simulink model "MCity_cs"  (Simulink 8.9)
settings: Solver=ode5  StartTime=0.0  StopTime=2.95  FixedStep=1/200  RelTol=1e-3
PreLoadFcn:
  | check_NUTS_defined;
  | 
  | assignin('base',['model_closed_' bdroot],false);
InitFcn:
  | PreScanExperimentInitFcn(bdroot)
StopFcn:
  | PreScanExperimentStopFcn(bdroot)
values from neighbouring files (symbols this model uses):
  d_offset = -18.15    [monocityTestLeftTurn.mat]    (also in simulation_leftTurn_PreScan.m = dl/vl*vh - 43 + R)
undefined symbols (not defined in the file or in its folder): DiscIntNeverNeededParam, warningInitialVelocity, x0
libraries: simulink x73, PreScanSimulinkLibrary x14, simulink_extras x10, PreScanUsefulBlocks x4
(part 9 of 11)

== system MCity_cs/BMW_Z3_1/Dynamics_Simple/Chassis/Bicycle_model_[XYZ]/Y & Yaw_Motion ==
  |vx|_[ms-1] : Inport
  Fy_[N] : Inport  Port=2
  Mz_[Nm] : Inport  Port=3
  Compare To Zero : simulink/Logic and Bit Operations/Compare To Zero  relop===  OutDataTypeStr=boolean  ZeroCross=off
  Configurable Subsystem : Subsystem  BlockChoice=Integrator  mask{ComputationMode=ComputationMode}
      mask prompts: ComputationMode "Computation mode:"
      mask init:
      | SetComputationMode(gcb,ComputationMode);
      settings: AttributesFormatString=%<BlockChoice>  OpenFcn=BringToFront(gcb);  MemberBlocks=Discrete-Time Integrator,Integrator
      settings: TemplateBlock=|
      | PreScanSimulinkLibrary/Configurable Subsystems/integral with reset/Configurable
      | Subsystem
  Configurable Subsystem1 : Subsystem  BlockChoice=Integrator  mask{ComputationMode=ComputationMode}
      link override Discrete-Time Integrator: IntegratorMethod=Integration: Backward Euler
      mask prompts: ComputationMode "Computation mode:"
      mask init:
      | SetComputationMode(gcb,ComputationMode);
      settings: AttributesFormatString=%<BlockChoice>  OpenFcn=BringToFront(gcb);  MemberBlocks=Discrete-Time Integrator,Integrator
      settings: TemplateBlock=|
      | PreScanSimulinkLibrary/Configurable Subsystems/integral/Configurable
      | Subsystem1
  Configurable Subsystem2 : Subsystem  BlockChoice=Integrator  mask{ComputationMode=ComputationMode}
      mask prompts: ComputationMode "Computation mode:"
      mask init:
      | SetComputationMode(gcb,ComputationMode);
      settings: AttributesFormatString=%<BlockChoice>  OpenFcn=BringToFront(gcb);  MemberBlocks=Discrete-Time Integrator,Integrator
      settings: TemplateBlock=|
      | PreScanSimulinkLibrary/Configurable Subsystems/integral with reset/Configurable
      | Subsystem
  Fcn1 : Fcn  Expr=u(1)*u(3)
  Gain : Gain  Gain=1/p.m  SaturateOnIntegerOverflow=on  OutDataTypeStr=Inherit: Same as input  ParamDataTypeStr=Inherit: Same as input
  Gain1 : Gain  Gain=1/p.J_zz  SaturateOnIntegerOverflow=on  OutDataTypeStr=Inherit: Same as input  ParamDataTypeStr=Inherit: Same as input
  Sum1 : Sum  Inputs=-+  SaturateOnIntegerOverflow=on  InputSameDT=on  OutDataTypeStr=Inherit: Same as first input
  mux : Mux  Inputs=3
  |vx|_[ms-1]1 : Outport  InitialOutput=0
  vy_[ms-1] : Outport  Port=2  InitialOutput=0
  ay_[ms-2] : Outport  Port=3  InitialOutput=0
  dYawAngle_[rads-1] : Outport  Port=4  InitialOutput=0
  YawAngle_[rad] : Outport  Port=5  InitialOutput=0
  wires:
  Configurable Subsystem2/1(Out1) -> Configurable Subsystem1/1(In1), mux/3, dYawAngle_[rads-1]/1  "dYawAngle_[rads-1]"
  Configurable Subsystem/1(Out1) -> mux/2, vy_[ms-1]/1  "vy_[ms-1]"
  |vx|_[ms-1]/1 -> mux/1, |vx|_[ms-1]1/1, Compare To Zero/1  "|vx|_[ms-1]"
  mux/1 -> Fcn1/1  "|vx|_[ms-1]_vy_[ms-1]_dYawAngle_[rads-1]"
  Fcn1/1 -> Sum1/1  "|vx|*dYawAngle_[ms-2]"
  Sum1/1 -> Configurable Subsystem/1(In1)  "dvy_[ms-2]"
  Fy_[N]/1 -> Gain/1  "Fy_[N]"
  Mz_[Nm]/1 -> Gain1/1  "Mz_[Nm]"
  Configurable Subsystem1/1(Out1) -> YawAngle_[rad]/1
  Compare To Zero/1 -> [reset]
  [reset] -> Configurable Subsystem2/2(In2)
  [reset] -> Configurable Subsystem/2(In2)
  Gain/1 -> ay_[ms-2]/1, Sum1/2  "ddy_[ms-2]"
  Gain1/1 -> Configurable Subsystem2/1(In1)  "ddYawAngle_[rads-2]"

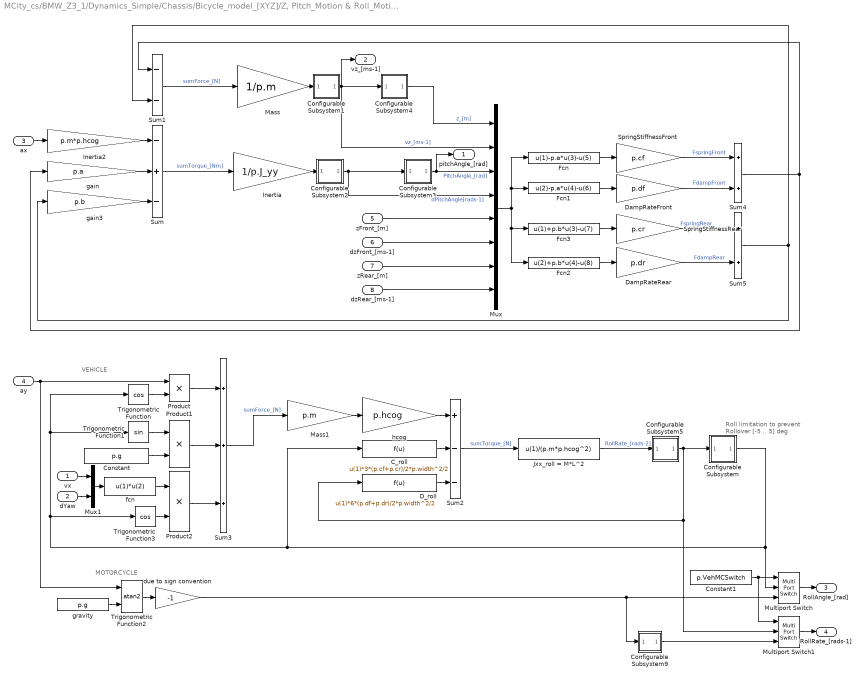
== system MCity_cs/BMW_Z3_1/Dynamics_Simple/Chassis/Bicycle_model_[XYZ]/Z, Pitch_Motion & Roll_Motion ==
  note: MOTORCYCLE
  note: VEHICLE
  note: Roll limitation
      | to prevent
      | Rollover
      | [-5 .. 5] deg
  vx : Inport
  dYaw : Inport  Port=2
  ax : Inport  Port=3
  ay : Inport  Port=4
  zFront_[m] : Inport  Port=5
  dzFront_[ms-1] : Inport  Port=6
  zRear_[m] : Inport  Port=7
  dzRear_[ms-1] : Inport  Port=8
  C_roll : Fcn  Expr=u(1)*3*(p.cf+p.cr)/2*p.width^2/2
  Configurable Subsystem : Subsystem  BlockChoice=Integrator  mask{ComputationMode=ComputationMode}
      link override Discrete-Time Integrator: UpperSaturationLimit=5*pi/180  LowerSaturationLimit=-5*pi/180
      link override Integrator: UpperSaturationLimit=5*pi/180  LowerSaturationLimit=-5*pi/180
      mask prompts: ComputationMode "Computation mode:"
      mask init:
      | SetComputationMode(gcb,ComputationMode);
      settings: AttributesFormatString=%<BlockChoice>  OpenFcn=BringToFront(gcb);  MemberBlocks=Discrete-Time Integrator,Integrator
      settings: TemplateBlock=|
      | PreScanSimulinkLibrary/Configurable Subsystems/integral with limits
      | for roll motion/Configurable
      | Subsystem
  Configurable Subsystem1 : Subsystem  BlockChoice=Integrator  mask{ComputationMode=ComputationMode}
      mask prompts: ComputationMode "Computation mode:"
      mask init:
      | SetComputationMode(gcb,ComputationMode);
      settings: AttributesFormatString=%<BlockChoice>  OpenFcn=BringToFront(gcb);  MemberBlocks=Discrete-Time Integrator,Integrator
      settings: TemplateBlock=|
      | PreScanSimulinkLibrary/Configurable Subsystems/integral/Configurable
      | Subsystem1
  Configurable Subsystem2 : Subsystem  BlockChoice=Integrator  mask{ComputationMode=ComputationMode}
      mask prompts: ComputationMode "Computation mode:"
      mask init:
      | SetComputationMode(gcb,ComputationMode);
      settings: AttributesFormatString=%<BlockChoice>  OpenFcn=BringToFront(gcb);  MemberBlocks=Discrete-Time Integrator,Integrator
      settings: TemplateBlock=|
      | PreScanSimulinkLibrary/Configurable Subsystems/integral/Configurable
      | Subsystem1
  Configurable Subsystem3 : Subsystem  BlockChoice=Integrator  mask{ComputationMode=ComputationMode}
      mask prompts: ComputationMode "Computation mode:"
      mask init:
      | SetComputationMode(gcb,ComputationMode);
      settings: AttributesFormatString=%<BlockChoice>  OpenFcn=BringToFront(gcb);  MemberBlocks=Discrete-Time Integrator,Integrator
      settings: TemplateBlock=|
      | PreScanSimulinkLibrary/Configurable Subsystems/integral/Configurable
      | Subsystem1
  Configurable Subsystem4 : Subsystem  BlockChoice=Integrator  mask{ComputationMode=ComputationMode}
      mask prompts: ComputationMode "Computation mode:"
      mask init:
      | SetComputationMode(gcb,ComputationMode);
      settings: AttributesFormatString=%<BlockChoice>  OpenFcn=BringToFront(gcb);  MemberBlocks=Discrete-Time Integrator,Integrator
      settings: TemplateBlock=|
      | PreScanSimulinkLibrary/Configurable Subsystems/integral/Configurable
      | Subsystem1
  Configurable Subsystem5 : Subsystem  BlockChoice=Integrator  mask{ComputationMode=ComputationMode}
      mask prompts: ComputationMode "Computation mode:"
      mask init:
      | SetComputationMode(gcb,ComputationMode);
      settings: AttributesFormatString=%<BlockChoice>  OpenFcn=BringToFront(gcb);  MemberBlocks=Discrete-Time Integrator,Integrator
      settings: TemplateBlock=|
      | PreScanSimulinkLibrary/Configurable Subsystems/integral/Configurable
      | Subsystem1
  Configurable Subsystem9 : Subsystem  BlockChoice=Derivative  mask{ComputationMode=ComputationMode}
      mask prompts: ComputationMode "Computation mode:"
      mask init:
      | SetComputationMode(gcb,ComputationMode);
      settings: AttributesFormatString=%<BlockChoice>  OpenFcn=BringToFront(gcb);  MemberBlocks=Derivative,Discrete Derivative
      settings: TemplateBlock=|
      | PreScanSimulinkLibrary/Configurable Subsystems/Derivative/Configurable
      | Subsystem
  Constant : Constant  Value=p.g
  Constant1 : Constant  Value=p.VehMCSwitch
  D_roll : Fcn  Expr=u(1)*6*(p.df+p.dr)/2*p.width^2/2
  DampRateFront : Gain  Gain=p.df  SaturateOnIntegerOverflow=on  OutDataTypeStr=Inherit: Same as input  ParamDataTypeStr=Inherit: Same as input
  DampRateRear : Gain  Gain=p.dr  SaturateOnIntegerOverflow=on  OutDataTypeStr=Inherit: Same as input  ParamDataTypeStr=Inherit: Same as input
  Fcn : Fcn  Expr=u(1)-p.a*u(3)-u(5)
  Fcn1 : Fcn  Expr=u(2)-p.a*u(4)-u(6)
  Fcn2 : Fcn  Expr=u(2)+p.b*u(4)-u(8)
  Fcn3 : Fcn  Expr=u(1)+p.b*u(3)-u(7)
  Inertia : Gain  Gain=1/p.J_yy  SaturateOnIntegerOverflow=on  OutDataTypeStr=Inherit: Same as input  ParamDataTypeStr=Inherit: Same as input
  Inertia2 : Gain  Gain=p.m*p.hcog  SaturateOnIntegerOverflow=on  OutDataTypeStr=Inherit: Same as input  ParamDataTypeStr=Inherit: Same as input
  Jxx_roll = M*L^2 : Fcn  Expr=u(1)/(p.m*p.hcog^2)
  Mass : Gain  Gain=1/p.m  SaturateOnIntegerOverflow=on  OutDataTypeStr=Inherit: Same as input  ParamDataTypeStr=Inherit: Same as input
  Mass1 : Gain  Gain=p.m  SaturateOnIntegerOverflow=on  OutDataTypeStr=Inherit: Same as input  ParamDataTypeStr=Inherit: Same as input
  Multiport Switch : MultiPortSwitch  Inputs=2
  Multiport Switch1 : MultiPortSwitch  Inputs=2
  Mux : Mux  Inputs=8
  Mux1 : Mux  Inputs=2
  Product : Product  RndMeth=Zero
  Product1 : Product  RndMeth=Zero
  Product2 : Product  RndMeth=Zero
  SpringStiffnessFront : Gain  Gain=p.cf  SaturateOnIntegerOverflow=on  OutDataTypeStr=Inherit: Same as input  ParamDataTypeStr=Inherit: Same as input
  SpringStiffnessRear : Gain  Gain=p.cr  SaturateOnIntegerOverflow=on  OutDataTypeStr=Inherit: Same as input  ParamDataTypeStr=Inherit: Same as input
  Sum : Sum  Inputs=-+-  SaturateOnIntegerOverflow=on  InputSameDT=on  OutDataTypeStr=Inherit: Same as first input
  Sum1 : Sum  Inputs=--  SaturateOnIntegerOverflow=on  InputSameDT=on  OutDataTypeStr=Inherit: Same as first input
  Sum2 : Sum  Inputs=+--  SaturateOnIntegerOverflow=on  InputSameDT=on  OutDataTypeStr=Inherit: Same as first input
  Sum3 : Sum  Inputs=+++  SaturateOnIntegerOverflow=on  InputSameDT=on  OutDataTypeStr=Inherit: Same as first input
  Sum4 : Sum  SaturateOnIntegerOverflow=on  InputSameDT=on  OutDataTypeStr=Inherit: Same as first input
  Sum5 : Sum  SaturateOnIntegerOverflow=on  InputSameDT=on  OutDataTypeStr=Inherit: Same as first input
  Trigonometric Function : Trigonometry  Operator=cos
  Trigonometric Function1 : Trigonometry
  Trigonometric Function2 : Trigonometry  Operator=atan2
  Trigonometric Function3 : Trigonometry  Operator=cos
  due to sign convention : Gain  Gain=-1  SaturateOnIntegerOverflow=on  OutDataTypeStr=Inherit: Same as input  ParamDataTypeStr=Inherit: Same as input
  fcn : Fcn  Expr=u(1)*u(2)
  gain : Gain  Gain=p.a  SaturateOnIntegerOverflow=on  OutDataTypeStr=Inherit: Same as input  ParamDataTypeStr=Inherit: Same as input
  gain3 : Gain  Gain=p.b  SaturateOnIntegerOverflow=on  OutDataTypeStr=Inherit: Same as input  ParamDataTypeStr=Inherit: Same as input
  gravity : Constant  Value=p.g
  hcog : Gain  Gain=p.hcog  SaturateOnIntegerOverflow=on  OutDataTypeStr=Inherit: Same as input  ParamDataTypeStr=Inherit: Same as input
  pitchAngle_[rad] : Outport
  vz_[ms-1] : Outport  Port=2
  RollAngle_[rad] : Outport  Port=3
  RollRate_[rads-1] : Outport  Port=4
  wires:
  Inertia/1 -> Configurable Subsystem2/1(In1)
  Configurable Subsystem2/1(Out1) -> Configurable Subsystem3/1(In1), Mux/4  "dPitchAngle[rads-1]"
  Mass/1 -> Configurable Subsystem1/1(In1)
  Configurable Subsystem1/1(Out1) -> Configurable Subsystem4/1(In1), Mux/2, vz_[ms-1]/1  "vz_[ms-1]"
  ax/1 -> Inertia2/1
  Inertia2/1 -> Sum/1
  zFront_[m]/1 -> Mux/5
  dzFront_[ms-1]/1 -> Mux/6
  zRear_[m]/1 -> Mux/7
  dzRear_[ms-1]/1 -> Mux/8
  Configurable Subsystem4/1(Out1) -> Mux/1  "z_[m]"
  SpringStiffnessFront/1 -> Sum4/1  "FspringFront"
  DampRateFront/1 -> Sum4/2  "FdampFront"
  DampRateRear/1 -> Sum5/2  "FdampRear"
  SpringStiffnessRear/1 -> Sum5/1  "FspringRear"
  gain3/1 -> Sum/3
  gain/1 -> Sum/2
  Configurable Subsystem3/1(Out1) -> Mux/3, pitchAngle_[rad]/1  "PitchAngle_[rad]"
  Sum4/1 -> Sum1/1, gain/1
  Sum5/1 -> gain3/1, Sum1/2
  Sum2/1 -> Jxx_roll = M*L^2/1  "sumTorque_[N]"
  Jxx_roll = M*L^2/1 -> Configurable Subsystem5/1(In1)  "RollRate_[rads-2]"
  Configurable Subsystem5/1(Out1) -> Configurable Subsystem/1(In1), D_roll/1, Multiport Switch1/2
  Configurable Subsystem/1(Out1) -> C_roll/1, Trigonometric Function1/1, Trigonometric Function/1, Trigonometric Function3/1, Multiport Switch/2
  Trigonometric Function/1 -> Product/2
  ay/1 -> Product/1, Trigonometric Function2/1
  Trigonometric Function1/1 -> Product1/1
  Constant/1 -> Product1/2
  Product/1 -> Sum3/1
  Product1/1 -> Sum3/2
  Mass1/1 -> hcog/1
  hcog/1 -> Sum2/1
  C_roll/1 -> Sum2/2
  D_roll/1 -> Sum2/3
  Mux/1 -> Fcn2/1, Fcn3/1, Fcn/1, Fcn1/1
  Fcn/1 -> SpringStiffnessFront/1
  Fcn1/1 -> DampRateFront/1
  Fcn3/1 -> SpringStiffnessRear/1
  Fcn2/1 -> DampRateRear/1
  due to sign convention/1 -> Configurable Subsystem9/1(In1), Multiport Switch/3
  Trigonometric Function2/1 -> due to sign convention/1
  gravity/1 -> Trigonometric Function2/2
  Constant1/1 -> Multiport Switch/1, Multiport Switch1/1
  Multiport Switch/1 -> RollAngle_[rad]/1
  Multiport Switch1/1 -> RollRate_[rads-1]/1
  Configurable Subsystem9/1(Out1) -> Multiport Switch1/3
  Mux1/1 -> fcn/1
  vx/1 -> Mux1/1
  dYaw/1 -> Mux1/2
  fcn/1 -> Product2/1
  Trigonometric Function3/1 -> Product2/2
  Product2/1 -> Sum3/3
  Sum/1 -> Inertia/1  "sumTorque_[Nm]"
  Sum1/1 -> Mass/1  "sumForce_[N]"
  Sum3/1 -> Mass1/1  "sumForce_[N]"

== system MCity_cs/BMW_Z3_1/Dynamics_Simple/Chassis/FrontTyre/AlphaFront ==
  In : Inport
  Abs : Abs
  Compare To Constant : simulink/Logic and Bit Operations/Compare To Constant  relop=>  const=0  OutDataTypeStr=uint8  ZeroCross=off
  Enabled Subsystem : Subsystem  TreatAsAtomicUnit=on
  Selector : Selector  IndexOptions=Index vector (dialog)  Indices=1  OutputSizes=1
  Alpha : Outport
  wires:
  Selector/1 -> Abs/1
  Compare To Constant/1 -> Enabled Subsystem/Enable
  Enabled Subsystem/1(Alpha) -> Alpha/1
  In/1 -> Enabled Subsystem/1(In), Selector/1
  Abs/1 -> Compare To Constant/1

== system MCity_cs/BMW_Z3_1/Dynamics_Simple/Chassis/FrontTyre/Configurable Subsystem ==
  In1 : Inport
  In2 : Inport  Port=2
  Integrator : Integrator  ExternalReset=level  LimitOutput=on  UpperSaturationLimit=1  LowerSaturationLimit=-1
  Out1 : Outport
  wires:
  In1/1 -> Integrator/1
  In2/1 -> Integrator/2
  Integrator/1 -> Out1/1

== system MCity_cs/BMW_Z3_1/Dynamics_Simple/Chassis/FrontTyre/Configurable Subsystem1 ==
  In1 : Inport
  In2 : Inport  Port=2
  Integrator : Integrator  ExternalReset=level
  Out1 : Outport
  wires:
  In1/1 -> Integrator/1
  In2/1 -> Integrator/2
  Integrator/1 -> Out1/1

== system MCity_cs/BMW_Z3_1/Dynamics_Simple/Chassis/FrontTyre/Prevent_instability_at_low_Vx ==
  note: |vx|
  alpha[rad] : Inport
  In : Inport  Port=2
  Divide : Product  Inputs=**
  Lookup Table : Lookup  InputValues="[0    2.5   ]"  Table="[0.01    1]"  LookUpMeth=Interpolation-Use End Values
  Selector : Selector  InputPortWidth=3  IndexOptions=Index vector (dialog)  Indices=[1]  OutputSizes=1
  alpha [rad] : Outport
  wires:
  In/1 -> Selector/1
  Lookup Table/1 -> Divide/2
  Selector/1 -> Lookup Table/1
  alpha[rad]/1 -> Divide/1
  Divide/1 -> alpha [rad]/1

== system MCity_cs/BMW_Z3_1/Dynamics_Simple/Chassis/MuxDynState/Configurable Subsystem1 ==
  In1 : Inport
  Integrator : Integrator
  Out1 : Outport
  wires:
  In1/1 -> Integrator/1
  Integrator/1 -> Out1/1

== system MCity_cs/BMW_Z3_1/Dynamics_Simple/Chassis/MuxDynState/Transformation_BODY2GLOBAL ==
  Vvector_BODY_[m/s] : Inport
  angles_BODYwrtGLOB_[rad] : Inport  Port=2
  Dot Product : DotProduct  InputSameDT=on  OutDataTypeStr=Inherit: Inherit via internal rule
  Dot Product1 : DotProduct  InputSameDT=on  OutDataTypeStr=Inherit: Inherit via internal rule
  Dot Product2 : DotProduct  InputSameDT=on  OutDataTypeStr=Inherit: Inherit via internal rule
  Fcn10 : Fcn  Expr=cos(u(1))*sin(u(2))*sin(u(3))-sin(u(1))*cos(u(3))
  Fcn11 : Fcn  Expr=cos(u(1))*sin(u(2))*cos(u(3))+sin(u(1))*sin(u(3))
  Fcn12 : Fcn  Expr=sin(u(1))*cos(u(2))
  Fcn13 : Fcn  Expr=sin(u(1))*sin(u(2))*sin(u(3))+cos(u(1))*cos(u(3))
  Fcn14 : Fcn  Expr=sin(u(1))*sin(u(2))*cos(u(3))-cos(u(1))*sin(u(3))
  Fcn15 : Fcn  Expr=-sin(u(2))
  Fcn16 : Fcn  Expr=cos(u(2))*sin(u(3))
  Fcn17 : Fcn  Expr=cos(u(2))*cos(u(3))
  Fcn9 : Fcn  Expr=cos(u(1))*cos(u(2))
  Mux1 : Mux  Inputs=9
  Mux3 : Mux  Inputs=3
  Selector : Selector  InputPortWidth=9  IndexOptions=Index vector (dialog)  Indices=[1 2 3]  OutputSizes=1
  Selector1 : Selector  InputPortWidth=9  IndexOptions=Index vector (dialog)  Indices=[4 5 6]  OutputSizes=1
  Selector2 : Selector  InputPortWidth=9  IndexOptions=Index vector (dialog)  Indices=[7 8 9]  OutputSizes=1
  rot_xyz 2 rot_zyx : Selector  InputPortWidth=3  IndexOptions=Index vector (dialog)  Indices=[3 2 1]  OutputSizes=1
  Vvector_GLOBAL_[m/s] : Outport
  wires:
  Fcn9/1 -> Mux1/1
  Fcn10/1 -> Mux1/2
  Fcn11/1 -> Mux1/3
  Fcn12/1 -> Mux1/4
  Fcn13/1 -> Mux1/5
  Fcn14/1 -> Mux1/6
  Fcn15/1 -> Mux1/7
  Fcn16/1 -> Mux1/8
  Fcn17/1 -> Mux1/9
  Mux1/1 -> Selector/1, Selector1/1, Selector2/1  "RotationMatrix Visu"
  Selector/1 -> Dot Product/2
  Vvector_BODY_[m/s]/1 -> Dot Product2/1, Dot Product1/1, Dot Product/1
  Dot Product/1 -> Mux3/1
  Selector1/1 -> Dot Product1/2
  Selector2/1 -> Dot Product2/2
  Dot Product2/1 -> Mux3/3
  Dot Product1/1 -> Mux3/2
  rot_xyz 2 rot_zyx/1 -> Fcn9/1, Fcn10/1, Fcn11/1, Fcn12/1, Fcn13/1, Fcn14/1, Fcn15/1, Fcn16/1, Fcn17/1
  Mux3/1 -> Vvector_GLOBAL_[m/s]/1
  angles_BODYwrtGLOB_[rad]/1 -> rot_xyz 2 rot_zyx/1

== system MCity_cs/BMW_Z3_1/Dynamics_Simple/Chassis/RearTyre/AlphaRear ==
  In : Inport
  Abs : Abs
  Compare To Constant : simulink/Logic and Bit Operations/Compare To Constant  relop=>  const=0  OutDataTypeStr=uint8  ZeroCross=off
  Enabled Subsystem : Subsystem  TreatAsAtomicUnit=on
  Selector : Selector  IndexOptions=Index vector (dialog)  Indices=1  OutputSizes=1
  Alpha : Outport
  wires:
  Selector/1 -> Abs/1
  Compare To Constant/1 -> Enabled Subsystem/Enable
  Enabled Subsystem/1(Alpha) -> Alpha/1
  In/1 -> Enabled Subsystem/1(In), Selector/1
  Abs/1 -> Compare To Constant/1

== system MCity_cs/BMW_Z3_1/Dynamics_Simple/Chassis/RearTyre/Configurable Subsystem ==
  In1 : Inport
  In2 : Inport  Port=2
  Integrator : Integrator  ExternalReset=level
  Out1 : Outport
  wires:
  In1/1 -> Integrator/1
  In2/1 -> Integrator/2
  Integrator/1 -> Out1/1

== system MCity_cs/BMW_Z3_1/Dynamics_Simple/Chassis/RearTyre/Configurable Subsystem1 ==
  In1 : Inport
  In2 : Inport  Port=2
  Integrator : Integrator  ExternalReset=level  LimitOutput=on  UpperSaturationLimit=1  LowerSaturationLimit=-1
  Out1 : Outport
  wires:
  In1/1 -> Integrator/1
  In2/1 -> Integrator/2
  Integrator/1 -> Out1/1

== system MCity_cs/BMW_Z3_1/Dynamics_Simple/ShiftLogic/Detect Increase/If V0 higher of the from 2->3 shifting velocity ==
  In1 : Inport
  Action Port : ActionPort  PropagateVarSize=During execution  ActionType=then
  Out1 : Outport
  wires:
  In1/1 -> Out1/1

== system MCity_cs/BMW_Z3_1/Dynamics_Simple/ShiftLogic/Detect Increase/Other ==
  In1 : Inport
  Action Port : ActionPort  PropagateVarSize=During execution  ActionType=else
  Data Type Conversion : DataTypeConversion  OutDataTypeStr=double
  Detect Increase : simulink/Logic and Bit Operations/Detect Increase  vinit=0.0  InputProcessing=Inherited  OutDataTypeStr=uint8
  Out1 : Outport
  wires:
  In1/1 -> Detect Increase/1
  Detect Increase/1 -> Data Type Conversion/1
  Data Type Conversion/1 -> Out1/1

== system MCity_cs/BMW_Z3_1/Dynamics_Simple/Transmission/Transmission_Ratio/If Action Neutral ==
  In1 : Inport
  Action Port : ActionPort  InitializeStates=reset  PropagateVarSize=During execution  ActionType=then
  Out1 : Outport
  wires:
  In1/1 -> Out1/1

== system MCity_cs/BMW_Z3_1/Dynamics_Simple/Transmission/Transmission_Ratio/If Action Normal ==
  In1 : Inport
  Action Port : ActionPort  InitializeStates=reset  PropagateVarSize=During execution  ActionType=else
  Out1 : Outport
  wires:
  In1/1 -> Out1/1

== system MCity_cs/BMW_Z3_1/Dynamics_Simple/Transmission/Transmission_Ratio/If Action Reverse ==
  In1 : Inport
  Action Port : ActionPort  InitializeStates=reset  PropagateVarSize=During execution  ActionType=elseif
  Reverse : Gain  Gain=-1
  Out1 : Outport
  wires:
  Reverse/1 -> Out1/1
  In1/1 -> Reverse/1

== system MCity_cs/BMW_Z3_1/PathFollower_Preview_1/LateralController/CTRL REFERENCES/Calculate Lateral Error ==
  In1 : Inport
  In2 : Inport  Port=2
  In3 : Inport  Port=3
  In4 : Inport  Port=4
  In5 : Inport  Port=5
  eml_find_10k_lateral_error_points : MATLAB Function  TreatAsAtomicUnit=on
  Out1 : Outport
  wires:
  In5/1 -> eml_find_10k_lateral_error_points/5(PreviewDistance)
  In4/1 -> eml_find_10k_lateral_error_points/4(p0)
  eml_find_10k_lateral_error_points/1(dist_psvehicle) -> Out1/1
  In3/1 -> eml_find_10k_lateral_error_points/3(ActorOffset_Left_Right)
  In2/1 -> eml_find_10k_lateral_error_points/2(TrajOffset_x_y_Y)
  In1/1 -> eml_find_10k_lateral_error_points/1(pvp)

== system MCity_cs/BMW_Z3_1/PathFollower_Preview_1/LateralController/CTRL REFERENCES/Calculate Preview Point (pvp) by extrapolating current Vehicle Position (p0) with Preview Distance and Vehicle Orientation ==
  Preview Distance : Inport
  x,y,Y Demux [m,m,rad] : Inport  Port=2
  Fcn : Fcn  Expr=u(2)*cos(u(1))
  Fcn1 : Fcn  Expr=u(2)*sin(u(1))
  Mux : Mux  Inputs=2
  Selector1 : Selector  InputPortWidth=3  IndexOptions=Index vector (dialog)  Indices=[1]  OutputSizes=1
  Selector2 : Selector  InputPortWidth=3  IndexOptions=Index vector (dialog)  Indices=[2]  OutputSizes=1
  Selector3 : Selector  InputPortWidth=3  IndexOptions=Index vector (dialog)  Indices=[3]  OutputSizes=1
  Sum : Sum  Inputs=|++
  Sum1 : Sum  Inputs=|++
  x_glob_PVP : Outport
  y_glob_PVP : Outport  Port=2
  Y [rad] : Outport  Port=3
  wires:
  Selector3/1 -> Mux/1, Y [rad]/1
  Selector1/1 -> Sum/1
  Selector2/1 -> Sum1/1
  Preview Distance/1 -> Mux/2
  Mux/1 -> Fcn/1, Fcn1/1
  Fcn/1 -> Sum/2
  Fcn1/1 -> Sum1/2
  Sum/1 -> x_glob_PVP/1
  Sum1/1 -> y_glob_PVP/1
  x,y,Y Demux [m,m,rad]/1 -> Selector2/1, Selector1/1, Selector3/1

== system MCity_cs/BMW_Z3_1/PathFollower_Preview_1/LateralController/CTRL REFERENCES/Find Reference Point (pref0) on Trajectory closest to P0 Point (p0) ==
  In1 : Inport
  In2 : Inport  Port=2
  In3 : Inport  Port=3
  In4 : Inport  Port=4
  eml_find_closest_trajectory_points0 : MATLAB Function  TreatAsAtomicUnit=on
  Out1 : Outport
  Out2 : Outport  Port=2
  wires:
  eml_find_closest_trajectory_points0/2(Actor_traj_angle) -> Out2/1
  eml_find_closest_trajectory_points0/1(Actor_traj_distance) -> Out1/1
  In4/1 -> eml_find_closest_trajectory_points0/4(p0)
  In3/1 -> eml_find_closest_trajectory_points0/3(ActorOffset_Left_Right)
  In2/1 -> eml_find_closest_trajectory_points0/2(TrajOffset_x_y_Y)
  In1/1 -> eml_find_closest_trajectory_points0/1(pvp)

== system MCity_cs/BMW_Z3_1/PathFollower_Preview_1/LateralController/SteeringWheelAngle/FirstOrderDynamics ==
  In : Inport
  TimeConstant[s] : Inport  Port=2
  Reset : Inport  Port=3
  x0 : Inport  Port=4
  1|TimeConstant : Product  Inputs=*/  SaturateOnIntegerOverflow=on  InputSameDT=on  OutDataTypeStr=Inherit: Same as first input
  Discrete-Time Integrator : DiscreteIntegrator  ExternalReset=rising  InitialConditionSource=external  InitialCondition=x0  SampleTime=CSSampleTime  ICPrevOutput=DiscIntNeverNeededParam  ICPrevScaledInput=DiscIntNeverNeededParam
  IC : InitialCondition  Value=0
  Saturation : Saturate  UpperLimit=1e300  LowerLimit=0.001
  Sum : Sum  Inputs=-+|  SaturateOnIntegerOverflow=on  InputSameDT=on  OutDataTypeStr=Inherit: Same as first input
  Out : Outport
  wires:
  IC/1 -> Discrete-Time Integrator/3
  In/1 -> Sum/2
  x0/1 -> IC/1
  Reset/1 -> Discrete-Time Integrator/2
  1|TimeConstant/1 -> Discrete-Time Integrator/1
  Sum/1 -> 1|TimeConstant/1
  Saturation/1 -> 1|TimeConstant/2
  TimeConstant[s]/1 -> Saturation/1
  Discrete-Time Integrator/1 -> Out/1, Sum/1

== system MCity_cs/BMW_Z3_1/PathFollower_Preview_1/LateralController/SteeringWheelAngle/Sat_Total ==
  In : Inport
  Sat_Limit : Inport  Port=2
  Gain1 : Gain  Gain=-1  SaturateOnIntegerOverflow=on  OutDataTypeStr=Inherit: Same as input  ParamDataTypeStr=Inherit: Same as input
  RelOp_UL : RelationalOperator  RndMeth=Nearest
  RelOp_UL1 : RelationalOperator  Operator=<=  RndMeth=Nearest
  Sum : Sum  Inputs=++|  SaturateOnIntegerOverflow=on
  Switch : Switch  Threshold=0.5  SaturateOnIntegerOverflow=on
  Switch1 : Switch  Threshold=0.5  SaturateOnIntegerOverflow=on
  Sat_Total : Outport
  Sat_Info : Outport  Port=2
  wires:
  Sat_Limit/1 -> Gain1/1, Switch/1, RelOp_UL/2
  RelOp_UL/1 -> Switch/2, Sum/2
  Switch/1 -> RelOp_UL1/1, Switch1/3
  Gain1/1 -> RelOp_UL1/2, Switch1/1
  RelOp_UL1/1 -> Switch1/2, Sum/1
  In/1 -> Switch/3, RelOp_UL/1
  Switch1/1 -> Sat_Total/1
  Sum/1 -> Sat_Info/1

== system MCity_cs/BMW_Z3_1/PathFollower_Preview_1/LongitudinalController/If Desired Velocity ~= 0/PID Controller ==
  e : Inport
  Derivative Gain : Gain  Gain=D  SaturateOnIntegerOverflow=on  OutDataTypeStr=Inherit: Same as input  ParamDataTypeStr=Inherit: Same as input
  Discrete-Time Integrator : DiscreteIntegrator  gainval=1  SampleTime=CSSampleTime  ICPrevOutput=DiscIntNeverNeededParam  ICPrevScaledInput=DiscIntNeverNeededParam
  Filter : DiscreteIntegrator  gainval=1  SampleTime=CSSampleTime  ICPrevOutput=DiscIntNeverNeededParam  ICPrevScaledInput=DiscIntNeverNeededParam
  Integral Gain : Gain  Gain=I  SaturateOnIntegerOverflow=on  OutDataTypeStr=Inherit: Same as input  ParamDataTypeStr=Inherit: Same as input
  Proportional Gain : Gain  Gain=P  SaturateOnIntegerOverflow=on  OutDataTypeStr=Inherit: Same as input  ParamDataTypeStr=Inherit: Same as input
  Sum : Sum  Inputs=+++  SaturateOnIntegerOverflow=on  InputSameDT=on  OutDataTypeStr=Inherit: Same as first input
  Sum1 : Sum  Inputs=|+-  SaturateOnIntegerOverflow=on  InputSameDT=on  OutDataTypeStr=Inherit: Same as first input
  u : Outport  InitialOutput=0
  wires:
  Sum1/1 -> Filter/1, Sum/3
  Filter/1 -> Sum1/2
  Derivative Gain/1 -> Sum1/1
  Sum/1 -> u/1
  e/1 -> Integral Gain/1, Proportional Gain/1, Derivative Gain/1
  Discrete-Time Integrator/1 -> Sum/2
  Proportional Gain/1 -> Sum/1
  Integral Gain/1 -> Discrete-Time Integrator/1

== system MCity_cs/BMW_Z3_1/Subsystem/PreBraking Model/Bend road segment/Lead Car Longitudinal Velocity ==
  note: === TIS1 Lead Car Longitudinal Velocity block ===
      |
      |  - computes relative velocity between the EGO and leading car.
  TIS1 Rangedot [m/s] : Inport
  theta [rad] : Inport  Port=2
  lambda [rad] : Inport  Port=3
  Add1 : Sum  Inputs=+-
  Constant : Constant  Value=0
  Divide2 : Product  Inputs=*/
  Switch1 : Switch  Criteria=u2 ~= 0
  TIS1 Rangedot [m/s]1 : InportShadow
  Trigonometric Function : Trigonometry  Operator=cos
  Vw [m/s] : Outport
  wires:
  TIS1 Rangedot [m/s]/1 -> Divide2/1
  lambda [rad]/1 -> Add1/1
  theta [rad]/1 -> Add1/2
  Add1/1 -> Trigonometric Function/1
  Trigonometric Function/1 -> Divide2/2
  Divide2/1 -> Switch1/1
  Switch1/1 -> Vw [m/s]/1
  TIS1 Rangedot [m/s]1/1 -> Switch1/2
  Constant/1 -> Switch1/3

== system MCity_cs/BMW_Z3_1/Subsystem/PreBraking Model/Bend road segment/Lead Car Longitudinal Velocity1 ==
  note: === TIS1 Lead Car Longitudinal Velocity block ===
      |
      |  - computes relative velocity between the EGO and leading car.
  TIS2 Rangedot [m/s] : Inport
  theta [rad] : Inport  Port=2
  lambda [rad] : Inport  Port=3
  Add1 : Sum  Inputs=+-
  Constant : Constant  Value=0
  Divide2 : Product  Inputs=*/
  Switch1 : Switch  Criteria=u2 ~= 0
  TIS1 Rangedot [m/s]1 : InportShadow
  Trigonometric Function : Trigonometry  Operator=cos
  Vw [m/s] : Outport
  wires:
  TIS2 Rangedot [m/s]/1 -> Divide2/1
  lambda [rad]/1 -> Add1/1
  theta [rad]/1 -> Add1/2
  Add1/1 -> Trigonometric Function/1
  Trigonometric Function/1 -> Divide2/2
  Divide2/1 -> Switch1/1
  Switch1/1 -> Vw [m/s]/1
  TIS1 Rangedot [m/s]1/1 -> Switch1/2
  Constant/1 -> Switch1/3

== system MCity_cs/BMW_Z3_1/Subsystem/PreBraking Model/Bend road segment/T0.6 ==
  note: === T1.6 block ==
      |
      |    - compare TTC and output adequate binary vector flag.
  TTC : Inport
  Constant TTC : Inport  Port=2
  Gain : Gain  Gain=2
  Gain1 : Gain  Gain=ones(TISdet(2),1)
  Relational Operator1 : RelationalOperator  Operator=<  OutDataTypeStr=fixdt(1,16)  RndMeth=Nearest
  Switch : Switch  Criteria=u2 > Threshold
  all_flags_0.6 : Outport
  wires:
  Switch/1 -> Relational Operator1/1
  Relational Operator1/1 -> all_flags_0.6/1
  TTC/1 -> Switch/2, Switch/1
  Gain/1 -> Switch/3
  Constant TTC/1 -> Gain1/1
  Gain1/1 -> Gain/1, Relational Operator1/2

== system MCity_cs/BMW_Z3_1/Subsystem/PreBraking Model/Bend road segment/T1.6 ==
  note: === T1.6 block ==
      |
      |    - compare TTC and output adequate binary vector flag.
  TTC : Inport
  Constant TTC : Inport  Port=2
  Gain : Gain  Gain=2
  Gain1 : Gain  Gain=ones(TISdet(1),1)
  Relational Operator1 : RelationalOperator  Operator=<  OutDataTypeStr=fixdt(1,16)  RndMeth=Nearest
  Switch : Switch  Criteria=u2 > Threshold
  median filter : Subsystem
  all_flags_1.6 : Outport
  wires:
  Switch/1 -> Relational Operator1/1
  Relational Operator1/1 -> median filter/1(Flag in)
  TTC/1 -> Switch/2, Switch/1
  Gain/1 -> Switch/3
  Constant TTC/1 -> Gain1/1
  Gain1/1 -> Gain/1, Relational Operator1/2
  median filter/1(Flag out) -> all_flags_1.6/1

== system MCity_cs/BMW_Z3_1/Subsystem/PreBraking Model/Bend road segment/T2.6 ==
  note: === T1.6 block ==
      |
      |    - compare TTC and output adequate binary vector flag.
  TTC : Inport
  Constant TTC : Inport  Port=2
  Gain : Gain  Gain=2
  Gain1 : Gain  Gain=ones(TISdet(1),1)
  Relational Operator1 : RelationalOperator  Operator=<  OutDataTypeStr=fixdt(1,16)  RndMeth=Nearest
  Switch : Switch  Criteria=u2 > Threshold
  median filter : Subsystem
  all_flags_2.6 : Outport
  wires:
  Switch/1 -> Relational Operator1/1
  Relational Operator1/1 -> median filter/1(Flag in)
  TTC/1 -> Switch/2, Switch/1
  Gain/1 -> Switch/3
  Constant TTC/1 -> Gain1/1
  Gain1/1 -> Gain/1, Relational Operator1/2
  median filter/1(Flag out) -> all_flags_2.6/1

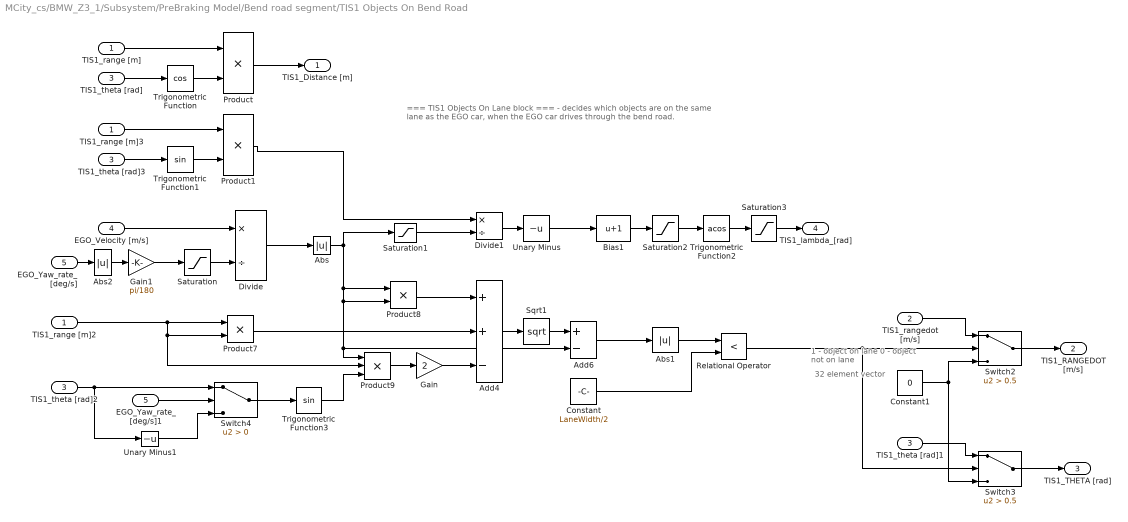
== system MCity_cs/BMW_Z3_1/Subsystem/PreBraking Model/Bend road segment/TIS1 Objects On Bend Road ==
  note: 1  - object      on lane
      | 0 - object not on lane
  note: 32 element vector
  note: === TIS1 Objects On Lane block ===
      |
      |  - decides which objects are on the same lane as the EGO car,
      |     when the EGO car drives through the bend road.
  TIS1_range [m] : Inport
  TIS1_rangedot [m/s] : Inport  Port=2
  TIS1_theta [rad] : Inport  Port=3
  EGO_Velocity [m/s] : Inport  Port=4
  EGO_Yaw_rate_[deg/s] : Inport  Port=5
  Abs : Abs
  Abs1 : Abs
  Abs2 : Abs
  Add4 : Sum  Inputs=++-
  Add6 : Sum  Inputs=+-
  Bias1 : Bias  Bias=1
  Constant : Constant  Value=LaneWidth/2
  Constant1 : Constant  Value=0
  Divide : Product  Inputs=*/
  Divide1 : Product  Inputs=*/
  EGO_Yaw_rate_[deg/s]1 : InportShadow  Port=5
  Gain : Gain  Gain=2
  Gain1 : Gain  Gain=pi/180
  Product{,1,7..8} (4 alike) : Product  RndMeth=Zero
  Product9 : Product  Inputs=3  RndMeth=Zero
  Relational Operator : RelationalOperator  Operator=<  OutDataTypeStr=boolean  RndMeth=Nearest
  Saturation : Saturate  UpperLimit=inf  LowerLimit=1e-6
  Saturation1 : Saturate  UpperLimit=inf  LowerLimit=1e-6
  Saturation2 : Saturate  UpperLimit=1  LowerLimit=-1
  Saturation3 : Saturate  UpperLimit=pi  LowerLimit=0
  Sqrt1 : Math  Operator=sqrt  SaturateOnIntegerOverflow=on
  Switch2 : Switch  Criteria=u2 > Threshold  Threshold=0.5
  Switch3 : Switch  Criteria=u2 > Threshold  Threshold=0.5
  Switch4 : Switch  Criteria=u2 > Threshold
  TIS1_range [m]2 : InportShadow
  TIS1_range [m]3 : InportShadow
  TIS1_theta [rad]1 : InportShadow  Port=3
  TIS1_theta [rad]2 : InportShadow  Port=3
  TIS1_theta [rad]3 : InportShadow  Port=3
  Trigonometric Function : Trigonometry  Operator=cos
  Trigonometric Function1 : Trigonometry
  Trigonometric Function2 : Trigonometry  Operator=acos
  Trigonometric Function3 : Trigonometry
  Unary Minus : UnaryMinus
  Unary Minus1 : UnaryMinus
  TIS1_Distance [m] : Outport
  TIS1_RANGEDOT [m/s] : Outport  Port=2
  TIS1_THETA [rad] : Outport  Port=3
  TIS1_lambda_[rad] : Outport  Port=4
  wires:
  TIS1_range [m]/1 -> Product/1
  TIS1_theta [rad]/1 -> Trigonometric Function/1
  Trigonometric Function/1 -> Product/2
  Trigonometric Function1/1 -> Product1/2
  EGO_Velocity [m/s]/1 -> Divide/1
  EGO_Yaw_rate_[deg/s]/1 -> Abs2/1
  Divide/1 -> Abs/1
  Relational Operator/1 -> Switch2/2, Switch3/2
  TIS1_rangedot [m/s]/1 -> Switch2/1
  TIS1_theta [rad]1/1 -> Switch3/1
  Constant1/1 -> Switch2/3, Switch3/3
  Switch2/1 -> TIS1_RANGEDOT [m/s]/1
  Switch3/1 -> TIS1_THETA [rad]/1
  Bias1/1 -> Saturation2/1
  Divide1/1 -> Unary Minus/1
  Unary Minus/1 -> Bias1/1
  Trigonometric Function2/1 -> Saturation3/1
  Abs/1 -> Product8/1, Product8/2, Product9/1, Add6/2, Saturation1/1
  Product/1 -> TIS1_Distance [m]/1
  Product8/1 -> Add4/1
  Product7/1 -> Add4/2
  Gain/1 -> Add4/3
  Product9/1 -> Gain/1
  Trigonometric Function3/1 -> Product9/3
  Add4/1 -> Sqrt1/1
  Sqrt1/1 -> Add6/1
  Add6/1 -> Abs1/1
  EGO_Yaw_rate_[deg/s]1/1 -> Switch4/2
  Switch4/1 -> Trigonometric Function3/1
  TIS1_theta [rad]2/1 -> Switch4/1, Unary Minus1/1
  Unary Minus1/1 -> Switch4/3
  TIS1_range [m]2/1 -> Product7/1, Product7/2, Product9/2
  TIS1_range [m]3/1 -> Product1/1
  TIS1_theta [rad]3/1 -> Trigonometric Function1/1
  Product1/1 -> Divide1/1
  Abs1/1 -> Relational Operator/1
  Constant/1 -> Relational Operator/2
  Saturation/1 -> Divide/2
  Saturation1/1 -> Divide1/2
  Saturation2/1 -> Trigonometric Function2/1
  Saturation3/1 -> TIS1_lambda_[rad]/1
  Gain1/1 -> Saturation/1
  Abs2/1 -> Gain1/1

== system MCity_cs/BMW_Z3_1/Subsystem/PreBraking Model/Bend road segment/TIS1 TTC Computing ==
  Distance [m] : Inport
  Velocity [m/s] : Inport  Port=2
  Compare : simulink/Logic and Bit Operations/Compare To Constant  relop===  const=1e-6  OutDataTypeStr=uint8  ZeroCross=off
  Constant : Constant  Value=0
  Data Type Conversion : DataTypeConversion
  Product : Product  Inputs=*/  RndMeth=Zero
  Saturation : Saturate  UpperLimit=inf  LowerLimit=1e-6
  Switch : Switch  Criteria=u2 > Threshold
  Switch1 : Switch  Criteria=u2 > Threshold  Threshold=0.5
  TTC [s] : Outport
  wires:
  Velocity [m/s]/1 -> Switch/2, Switch/1
  Constant/1 -> Switch/3, Switch1/1
  Switch/1 -> Saturation/1
  Distance [m]/1 -> Product/1
  Saturation/1 -> Product/2, Compare/1
  Compare/1 -> Data Type Conversion/1
  Product/1 -> Switch1/3
  Switch1/1 -> TTC [s]/1
  Data Type Conversion/1 -> Switch1/2

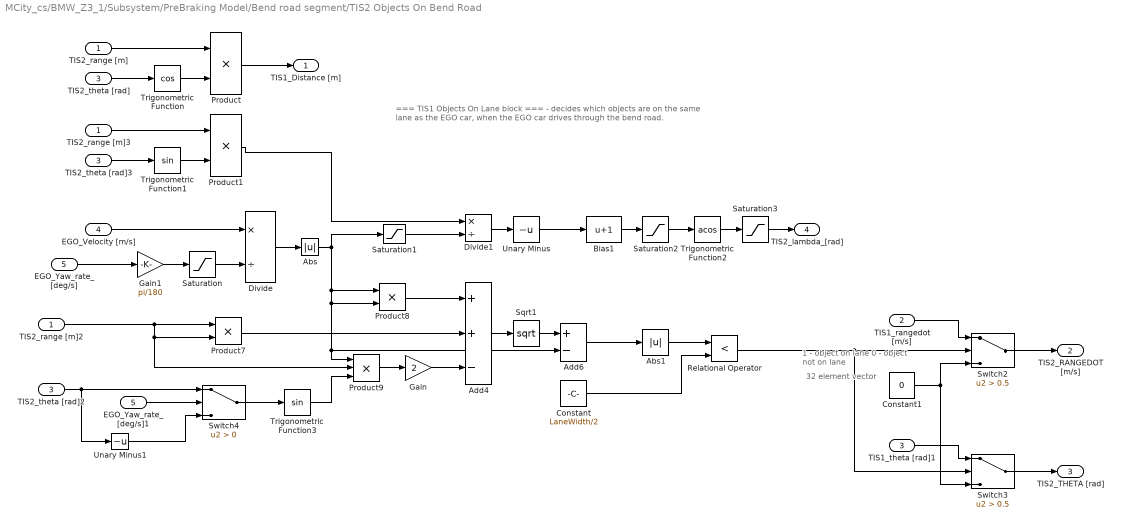
== system MCity_cs/BMW_Z3_1/Subsystem/PreBraking Model/Bend road segment/TIS2 Objects On Bend Road ==
  note: 1  - object      on lane
      | 0 - object not on lane
  note: 32 element vector
  note: === TIS1 Objects On Lane block ===
      |
      |  - decides which objects are on the same lane as the EGO car,
      |     when the EGO car drives through the bend road.
  TIS2_range [m] : Inport
  TIS1_rangedot [m/s] : Inport  Port=2
  TIS2_theta [rad] : Inport  Port=3
  EGO_Velocity [m/s] : Inport  Port=4
  EGO_Yaw_rate_[deg/s] : Inport  Port=5
  Abs : Abs
  Abs1 : Abs
  Add4 : Sum  Inputs=++-
  Add6 : Sum  Inputs=+-
  Bias1 : Bias  Bias=1
  Constant : Constant  Value=LaneWidth/2
  Constant1 : Constant  Value=0
  Divide : Product  Inputs=*/
  Divide1 : Product  Inputs=*/
  EGO_Yaw_rate_[deg/s]1 : InportShadow  Port=5
  Gain : Gain  Gain=2
  Gain1 : Gain  Gain=pi/180
  Product{,1,7..8} (4 alike) : Product  RndMeth=Zero
  Product9 : Product  Inputs=3  RndMeth=Zero
  Relational Operator : RelationalOperator  Operator=<  OutDataTypeStr=boolean  RndMeth=Nearest
  Saturation : Saturate  UpperLimit=inf  LowerLimit=1e-6
  Saturation1 : Saturate  UpperLimit=inf  LowerLimit=1e-6
  Saturation2 : Saturate  UpperLimit=1  LowerLimit=-1
  Saturation3 : Saturate  UpperLimit=pi  LowerLimit=0
  Sqrt1 : Math  Operator=sqrt  SaturateOnIntegerOverflow=on
  Switch2 : Switch  Criteria=u2 > Threshold  Threshold=0.5
  Switch3 : Switch  Criteria=u2 > Threshold  Threshold=0.5
  Switch4 : Switch  Criteria=u2 > Threshold
  TIS1_theta [rad]1 : InportShadow  Port=3
  TIS2_range [m]2 : InportShadow
  TIS2_range [m]3 : InportShadow
  TIS2_theta [rad]2 : InportShadow  Port=3
  TIS2_theta [rad]3 : InportShadow  Port=3
  Trigonometric Function : Trigonometry  Operator=cos
  Trigonometric Function1 : Trigonometry
  Trigonometric Function2 : Trigonometry  Operator=acos
  Trigonometric Function3 : Trigonometry
  Unary Minus : UnaryMinus
  Unary Minus1 : UnaryMinus
  TIS1_Distance [m] : Outport
  TIS2_RANGEDOT [m/s] : Outport  Port=2
  TIS2_THETA [rad] : Outport  Port=3
  TIS2_lambda_[rad] : Outport  Port=4
  wires:
  TIS2_range [m]/1 -> Product/1
  TIS2_theta [rad]/1 -> Trigonometric Function/1
  Trigonometric Function/1 -> Product/2
  Trigonometric Function1/1 -> Product1/2
  EGO_Velocity [m/s]/1 -> Divide/1
  EGO_Yaw_rate_[deg/s]/1 -> Gain1/1
  Divide/1 -> Abs/1
  Relational Operator/1 -> Switch2/2, Switch3/2
  TIS1_rangedot [m/s]/1 -> Switch2/1
  TIS1_theta [rad]1/1 -> Switch3/1
  Constant1/1 -> Switch2/3, Switch3/3
  Switch2/1 -> TIS2_RANGEDOT [m/s]/1
  Switch3/1 -> TIS2_THETA [rad]/1
  Bias1/1 -> Saturation2/1
  Divide1/1 -> Unary Minus/1
  Unary Minus/1 -> Bias1/1
  Trigonometric Function2/1 -> Saturation3/1
  Abs/1 -> Product8/1, Product8/2, Product9/1, Add6/2, Saturation1/1
  Product/1 -> TIS1_Distance [m]/1
  Product8/1 -> Add4/1
  Product7/1 -> Add4/2
  Gain/1 -> Add4/3
  Product9/1 -> Gain/1
  Trigonometric Function3/1 -> Product9/3
  Add4/1 -> Sqrt1/1
  Sqrt1/1 -> Add6/1
  Add6/1 -> Abs1/1
  EGO_Yaw_rate_[deg/s]1/1 -> Switch4/2
  Switch4/1 -> Trigonometric Function3/1
  TIS2_theta [rad]2/1 -> Unary Minus1/1, Switch4/1
  TIS2_range [m]2/1 -> Product7/1, Product7/2, Product9/2
  TIS2_range [m]3/1 -> Product1/1
  TIS2_theta [rad]3/1 -> Trigonometric Function1/1
  Product1/1 -> Divide1/1
  Abs1/1 -> Relational Operator/1
  Constant/1 -> Relational Operator/2
  Saturation/1 -> Divide/2
  Saturation1/1 -> Divide1/2
  Saturation2/1 -> Trigonometric Function2/1
  Saturation3/1 -> TIS2_lambda_[rad]/1
  Gain1/1 -> Saturation/1
  Unary Minus1/1 -> Switch4/3

== system MCity_cs/BMW_Z3_1/Subsystem/PreBraking Model/Bend road segment/TIS2 TTC Computing1 ==
  Distance [m] : Inport
  Velocity [m/s] : Inport  Port=2
  Compare : simulink/Logic and Bit Operations/Compare To Constant  relop===  const=1e-6  OutDataTypeStr=uint8  ZeroCross=off
  Constant : Constant  Value=0
  Data Type Conversion : DataTypeConversion
  Product : Product  Inputs=*/  RndMeth=Zero
  Saturation : Saturate  UpperLimit=inf  LowerLimit=1e-6
  Switch : Switch  Criteria=u2 > Threshold
  Switch1 : Switch  Criteria=u2 > Threshold  Threshold=0.5
  TTC [s] : Outport
  wires:
  Velocity [m/s]/1 -> Switch/2, Switch/1
  Constant/1 -> Switch/3, Switch1/1
  Switch/1 -> Saturation/1
  Distance [m]/1 -> Product/1
  Saturation/1 -> Product/2, Compare/1
  Compare/1 -> Data Type Conversion/1
  Product/1 -> Switch1/3
  Switch1/1 -> TTC [s]/1
  Data Type Conversion/1 -> Switch1/2

== system MCity_cs/BMW_Z3_1/Subsystem/PreBraking Model/Braking Lights/If Action Subsystem ==
  In1 : Inport
  Action Port : ActionPort  PropagateVarSize=During execution  ActionType=then
  Add : Sum
  Constant : Constant
  Unary Minus : UnaryMinus
  left light : Outport
  right light : Outport  Port=2
  wires:
  In1/1 -> left light/1, Unary Minus/1
  Add/1 -> right light/1
  Unary Minus/1 -> Add/1
  Constant/1 -> Add/2

== system MCity_cs/BMW_Z3_1/Subsystem/PreBraking Model/Display module/Display ==
  RPM : Inport
  V : Inport  Port=2
  BrakePressure : Inport  Port=3
  Throttle : Inport  Port=4
  Warning flag 2.6s : Inport  Port=5
  Enable : EnablePort  PropagateVarSize=During execution
  Brake Pressure [bar] : Gain  Gain=100/MaxBrakePressure
  DISPLAY : M-S-Function  FunctionName=msfcn_AEBS_PlotSpeed  Parameters=DisplayFreq DisplaySwitch
  Logical Operator1 : Logic  Operator=OR  Inputs=1  AllPortsSameDT=off  OutDataTypeStr=boolean
  Rounding Function{,1..3} (4 alike) : Rounding  Operator=round  SampleTime=1/DisplayFreq
  wires:
  Rounding Function/1 -> DISPLAY/1
  Rounding Function1/1 -> DISPLAY/2
  Rounding Function2/1 -> DISPLAY/3
  Rounding Function3/1 -> DISPLAY/4
  Brake Pressure [bar]/1 -> Rounding Function2/1
  Logical Operator1/1 -> DISPLAY/5
  RPM/1 -> Rounding Function/1
  V/1 -> Rounding Function1/1
  BrakePressure/1 -> Brake Pressure [bar]/1
  Throttle/1 -> Rounding Function3/1
  Warning flag 2.6s/1 -> Logical Operator1/1

== system MCity_cs/BMW_Z3_1/Subsystem/PreBraking Model/Interpretation/If Action Subsystem ==
  Action Port : ActionPort  PropagateVarSize=During execution  ActionType=then
  Constant : Constant
  Data Store Write : DataStoreWrite  DataStoreName=full
  wires:
  Constant/1 -> Data Store Write/1

== system MCity_cs/BMW_Z3_1/Subsystem/PreBraking Model/Interpretation/If Action Subsystem1 ==
  Action Port : ActionPort  PropagateVarSize=During execution  ActionType=then
  Constant : Constant
  Data Store Write : DataStoreWrite  DataStoreName=part
  wires:
  Constant/1 -> Data Store Write/1

== system MCity_cs/BMW_Z3_1/Subsystem/PreBraking Model/Interpretation/If Action Subsystem2 ==
  Action Port : ActionPort  PropagateVarSize=During execution  ActionType=then
  Constant : Constant  Value=0  SampleTime=min(Tsensor)
  Data Store Write : DataStoreWrite  DataStoreName=part
  wires:
  Constant/1 -> Data Store Write/1

== system MCity_cs/BMW_Z3_1/Subsystem/PreBraking Model/Radar/Radar ==
  TIS1 Range : Inport
  TIS1 Theta : Inport  Port=2
  TIS2 Range : Inport  Port=3
  TIS2 Theta : Inport  Port=4
  all_flags1.6 : Inport  Port=5
  all_flags2.6 : Inport  Port=6
  all_flags0.6 : Inport  Port=7
  Enable : EnablePort  PropagateVarSize=During execution
  Level-2 M-file S-Function : M-S-Function  FunctionName=msfcn_AEBS_radar_graph  Parameters=RadarFreq TISdet TISMaxRange TISMaxTheta RadarSwitch
  wires:
  TIS1 Range/1 -> Level-2 M-file S-Function/1
  TIS1 Theta/1 -> Level-2 M-file S-Function/2
  TIS2 Range/1 -> Level-2 M-file S-Function/3
  TIS2 Theta/1 -> Level-2 M-file S-Function/4
  all_flags1.6/1 -> Level-2 M-file S-Function/5
  all_flags2.6/1 -> Level-2 M-file S-Function/6
  all_flags0.6/1 -> Level-2 M-file S-Function/7

== system MCity_cs/BMW_Z3_1/Subsystem/PreBraking Model/Straight road segment/Impact point1 ==
  note: === Impact point block ===
      |
      |    - determines predicted distance to the point of impact,
      |    - passing through zero value, if there is no risk of collision.
  alfa : Inport
  xp [m] : Inport  Port=2
  yp [m] : Inport  Port=3
  Abs : Abs
  Add : Sum  Inputs=+-
  Compare To Constant : simulink/Logic and Bit Operations/Compare To Constant  relop=<  const=-1e-6  OutDataTypeStr=uint8  ZeroCross=off
  Compare To Constant1 : simulink/Logic and Bit Operations/Compare To Constant  relop=>  const=1e-6  OutDataTypeStr=uint8  ZeroCross=off
  Constant : Constant  Value=0
  Divide : Product  Inputs=*/
  Logical Operator : Logic  Operator=OR  AllPortsSameDT=off  OutDataTypeStr=boolean
  Saturation : Saturate  UpperLimit=inf  LowerLimit=1e-6
  Saturation1 : Saturate  UpperLimit=-1e-6  LowerLimit=-inf
  Saturation2 : Saturate  UpperLimit=300  LowerLimit=0
  Switch : Switch  Criteria=u2 > Threshold  Threshold=LaneWidth/2
  Switch1 : Switch  Criteria=u2 > Threshold  Threshold=0.5
  Switch2 : Switch  Criteria=u2 > Threshold
  Trigonometric Function : Trigonometry  Operator=tan
  xp [m]1 : InportShadow  Port=2
  yp [m]1 : InportShadow  Port=3
  xc [m] : Outport
  wires:
  yp [m]/1 -> Abs/1
  xp [m]/1 -> Switch/3
  Constant/1 -> Switch/1
  Switch/1 -> Switch1/3
  Abs/1 -> Switch/2
  xp [m]1/1 -> Add/1
  Divide/1 -> Add/2
  yp [m]1/1 -> Divide/1
  Trigonometric Function/1 -> Divide/2
  alfa/1 -> Compare To Constant1/1, Compare To Constant/1, Saturation1/1, Switch2/2, Saturation/1
  Compare To Constant1/1 -> Logical Operator/1
  Compare To Constant/1 -> Logical Operator/2
  Logical Operator/1 -> Switch1/2
  Switch1/1 -> Saturation2/1
  Add/1 -> Switch1/1
  Switch2/1 -> Trigonometric Function/1
  Saturation/1 -> Switch2/1
  Saturation1/1 -> Switch2/3
  Saturation2/1 -> xc [m]/1

== system MCity_cs/BMW_Z3_1/Subsystem/PreBraking Model/Straight road segment/Impact point2 ==
  note: === Impact point block ===
      |
      |    - determines predicted distance to the point of impact,
      |    - passing through zero value, if there is no risk of collision.
  alfa : Inport
  xp [m] : Inport  Port=2
  yp [m] : Inport  Port=3
  Abs : Abs
  Add : Sum  Inputs=+-
  Compare To Constant : simulink/Logic and Bit Operations/Compare To Constant  relop=<  const=-1e-6  OutDataTypeStr=uint8  ZeroCross=off
  Compare To Constant1 : simulink/Logic and Bit Operations/Compare To Constant  relop=>  const=1e-6  OutDataTypeStr=uint8  ZeroCross=off
  Constant : Constant  Value=0
  Divide : Product  Inputs=*/
  Logical Operator : Logic  Operator=OR  AllPortsSameDT=off  OutDataTypeStr=boolean
  Saturation : Saturate  UpperLimit=inf  LowerLimit=1e-6
  Saturation1 : Saturate  UpperLimit=-1e-6  LowerLimit=-inf
  Saturation2 : Saturate  UpperLimit=300  LowerLimit=0
  Switch : Switch  Criteria=u2 > Threshold  Threshold=LaneWidth/2
  Switch1 : Switch  Criteria=u2 > Threshold  Threshold=0.5
  Switch2 : Switch  Criteria=u2 > Threshold
  Trigonometric Function : Trigonometry  Operator=tan
  xp [m]1 : InportShadow  Port=2
  yp [m]1 : InportShadow  Port=3
  xc [m] : Outport
  wires:
  yp [m]/1 -> Abs/1
  xp [m]/1 -> Switch/3
  Constant/1 -> Switch/1
  Switch/1 -> Switch1/3
  Abs/1 -> Switch/2
  xp [m]1/1 -> Add/1
  Divide/1 -> Add/2
  yp [m]1/1 -> Divide/1
  Trigonometric Function/1 -> Divide/2
  alfa/1 -> Compare To Constant1/1, Compare To Constant/1, Saturation1/1, Switch2/2, Saturation/1
  Compare To Constant1/1 -> Logical Operator/1
  Compare To Constant/1 -> Logical Operator/2
  Logical Operator/1 -> Switch1/2
  Switch1/1 -> Saturation2/1
  Add/1 -> Switch1/1
  Switch2/1 -> Trigonometric Function/1
  Saturation/1 -> Switch2/1
  Saturation1/1 -> Switch2/3
  Saturation2/1 -> xc [m]/1

== system MCity_cs/BMW_Z3_1/Subsystem/PreBraking Model/Straight road segment/Relative velocity1 ==
  note: === Relative velocity block ===
      |
      |    - determines:
      |      -- relative, carthesian position of an obstacle,
      |      -- absolute values of carthesian velocity of an obstacle
      |          in respect to the actor orientation,
      |      -- relative velocity Vw beetwen actor and an obstacle
      |          in respect to actor front direction (x).
  V [m/s] : Inport
  range [m] : Inport  Port=2
  rangedot [m/s] : Inport  Port=3
  theta [rad] : Inport  Port=4
  theta_p [rad/s] : Inport  Port=5
  Abs{,1..3} (4 alike) : Abs
  Add : Sum  Inputs=++-
  Add2 : Sum  Inputs=-+
  Constant{,1..3} (4 alike) : Constant  Value=0
  Difference : simulink/Discrete/Difference  ICPrevInput=zeros(TISdet(1),1)  InputProcessing=Inherited  OutMin=[]  OutMax=[]  OutDataType=fixdt(1, 16)  OutScaling=2^-10  DoSatur=off
  Difference1 : simulink/Discrete/Difference  ICPrevInput=zeros(TISdet(1),1)  InputProcessing=Inherited  OutMin=[]  OutMax=[]  OutDataType=fixdt(1, 16)  OutScaling=2^-10  DoSatur=off
  Difference2 : simulink/Discrete/Difference  ICPrevInput=0.0  InputProcessing=Inherited  OutMin=[]  OutMax=[]  OutDataType=sfix(16)  OutScaling=2^-10  DoSatur=off
  Divide : Product  Inputs=**
  Divide1 : Product  Inputs=***
  Divide4 : Product  Inputs=**
  Divide6 : Product  Inputs=**
  Embedded MATLAB Function1 : MATLAB Function  TreatAsAtomicUnit=on
  Gain : Gain  Gain=0.01
  Saturation1 : Saturate  UpperLimit=50  LowerLimit=-50
  Saturation2 : Saturate  UpperLimit=150  LowerLimit=0
  Saturation3 : Saturate  UpperLimit=50  LowerLimit=-50
  Saturation4 : Saturate  UpperLimit=50  LowerLimit=-50
  Saturation5 : Saturate  UpperLimit=11.8  LowerLimit=-11.8
  Switch : Switch  Threshold=0.5
  Switch1 : Switch  Criteria=u2 > Threshold  Threshold=0.8
  Switch2 : Switch  Threshold=10
  Switch3 : Switch  Criteria=u2 > Threshold  Threshold=10
  Translation : MATLAB Function  TreatAsAtomicUnit=on
  Unit Delay : UnitDelay  InitialCondition=zeros(TISdet(1),50)  SampleTime=-1
  cos_theta : Trigonometry  Operator=cos
  sin_theta : Trigonometry
  yp' [m/s] : Outport
  xp' [m/s] : Outport  Port=2
  xp [m] : Outport  Port=3
  yp [m] : Outport  Port=4
  Vw [m/s] : Outport  Port=5
  wires:
  theta [rad]/1 -> cos_theta/1, sin_theta/1
  Divide/1 -> Saturation2/1
  range [m]/1 -> Divide/2, Divide6/1, Divide1/1, Embedded MATLAB Function1/1(r)
  sin_theta/1 -> Divide6/2, Divide1/2
  cos_theta/1 -> Divide/1, Divide4/1
  Divide6/1 -> Saturation5/1
  theta_p [rad/s]/1 -> Divide1/3
  Add2/1 -> Saturation3/1
  Divide4/1 -> Add2/1, Add/2
  Divide1/1 -> Add2/2, Add/3
  Saturation2/1 -> xp [m]/1
  Saturation5/1 -> Embedded MATLAB Function1/2(yp1), yp [m]/1
  Saturation1/1 -> Abs/1, Switch/1
  V [m/s]/1 -> Translation/1(v), Add/1
  Add/1 -> Saturation1/1
  Abs/1 -> Switch/2
  Constant/1 -> Switch/3
  Switch/1 -> Translation/2(xpd)
  Embedded MATLAB Function1/2(K2) -> Unit Delay/1
  Unit Delay/1 -> Embedded MATLAB Function1/3(K1)
  Embedded MATLAB Function1/1(yp2) -> Difference2/1
  Difference2/1 -> Gain/1
  Abs1/1 -> Switch1/2
  Constant1/1 -> Switch1/3
  Saturation4/1 -> yp' [m/s]/1
  Switch1/1 -> Difference/1, Switch2/3
  Switch2/1 -> Saturation4/1
  Difference/1 -> Abs2/1
  Abs2/1 -> Switch2/2
  Translation/1(xp_dot) -> Switch3/3, Difference1/1
  Abs3/1 -> Switch3/2
  Switch3/1 -> xp' [m/s]/1
  Constant2/1 -> Switch2/1
  Constant3/1 -> Switch3/1
  Difference1/1 -> Abs3/1
  rangedot [m/s]/1 -> Divide4/2
  Gain/1 -> Abs1/1, Switch1/1
  Saturation3/1 -> Vw [m/s]/1
